simulink model "lab4"  (R2018a)
settings: Solver=FixedStepDiscrete  StartTime=0  StopTime=0.2  RelTol=1e-3
libraries: powerlib x12, electricdrivelib x1
settings Model: Creator=Ali  LastModifiedBy=Ali

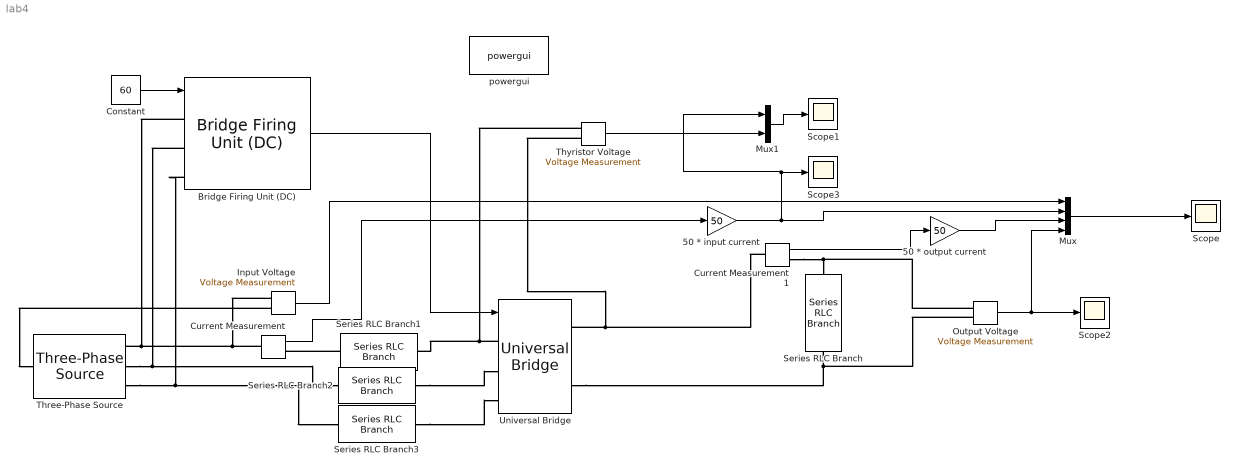
== system lab4 ==
  "50 * input current " : Gain  Gain=50
  50 * output current : Gain  Gain=50
  Bridge Firing Unit (DC) : electricdrivelib/Fundamental Drive Blocks/Bridge Firing Unit (DC)  OverrideUsingVariant=AC_Detailed_two quadrant  detailLevel=Detailed  nbPhases=3  numQuad=2  x4=50  x9=10  Ts=2e-6
      settings: SourceProductName=Simscape Power Systems  SourceProductBaseCode=PS
  Constant : Constant  Value=60
  Current Measurement : powerlib/Measurements/Current Measurement  PhasorSimulation=off  OutputType=Complex  PSBequivalent=0
  Current Measurement1 : powerlib/Measurements/Current Measurement  PhasorSimulation=off  OutputType=Complex  PSBequivalent=0
  Input Voltage : powerlib/Measurements/Voltage Measurement  PhasorSimulation=off  OutputType=Complex  PSBequivalent=0
  Mux : Mux
  Mux1 : Mux  Inputs=2
  Output Voltage : powerlib/Measurements/Voltage Measurement  PhasorSimulation=off  OutputType=Complex  PSBequivalent=0
  Scope{,1..3} (4 alike) : Scope
  Series RLC Branch : powerlib/Elements/Series RLC Branch  LConnTagsString=__new0  RConnTagsString=__new0  BranchType=RL  Resistance=72  Inductance=0.4575  SetiL0=off  InitialCurrent=0  Capacitance=1e-6  Setx0=off  InitialVoltage=0  Measurements=None
  Series RLC Branch1 : powerlib/Elements/Series RLC Branch  LConnTagsString=__new0  RConnTagsString=__new0  BranchType=L  Resistance=72  Inductance=5e-3  SetiL0=off  InitialCurrent=0  Capacitance=1e-6  Setx0=off  InitialVoltage=0  Measurements=None
  Series RLC Branch2 : powerlib/Elements/Series RLC Branch  LConnTagsString=__new0  RConnTagsString=__new0  BranchType=L  Resistance=72  Inductance=5e-3  SetiL0=off  InitialCurrent=0  Capacitance=1e-6  Setx0=off  InitialVoltage=0  Measurements=None
  Series RLC Branch3 : powerlib/Elements/Series RLC Branch  LConnTagsString=__new0  RConnTagsString=__new0  BranchType=L  Resistance=72  Inductance=5e-3  SetiL0=off  InitialCurrent=0  Capacitance=1e-6  Setx0=off  InitialVoltage=0  Measurements=None
  Three-Phase Source : powerlib/Electrical Sources/Three-Phase Source  InternalConnection=Yn  VoltagePhases=off  Voltage=347  PhaseAngle=0  Voltage_phases=[25e3 25e3 25e3]/sqrt(3)  PhaseAngles_phases=[0 -120 +120]  Frequency=50  NonIdealSource=on  SpecifyImpedance=off  Resistance=0  Inductance=0  ShortCircuitLevel=100e6  BaseVoltage=0  XRratio=7  BusType=swing  Pref=10e3  Qref=0  Prefabc=[10e3, 10e3, 10e3]  Qrefabc=[0, 0, 0]  Qmin=-inf  Qmax=inf
  Thyristor Voltage : powerlib/Measurements/Voltage Measurement  PhasorSimulation=off  OutputType=Complex  PSBequivalent=0
  Universal Bridge : powerlib/Power Electronics/Universal Bridge  Arms=3  SnubberResistance=1e5  SnubberCapacitance=inf  Device=Thyristors  Ron=1e-3  Lon=0  ForwardVoltages="[  0  0  ]"  ForwardVoltage=0  GTOparameters=[ 10e-6 , 20e-6 ]  IGBTparameters=[ 1e-6 , 2e-6 ]  Measurements=None  Measurements_2=None  converterType=Rectifier
  powergui : powerlib/powergui  Priority=1  SimulationMode=Discrete  SampleTime=50e-6  frequency=60  Iterations=50  frequencyindice=50  Pbase=100e6  ErrMax=1e-4  UnitsV=kV  UnitsW=MW  buscounter=0  FunctionMessages=off  echomessages=off  EnableUseOfTLC=off  CurrentSourceSwitches=off  DisableSnubberDevices=off  DisableRonSwitches=off  DisableVfSwitches=off  DisplayEquations=off  SolverType=Tustin/Backward Euler (TBE)  Interpol=off  ExternalGateDelay=off  methode=off  Ts=100  x0status=blocks  SPID=on  SwTol=0  HookPort=off  RestoreLinks=warning  ResistiveCurrentMeasurement=off  Frange=[0:2:500]  Ylog=off  Xlog=on  ShowGrid=off  save=off  variable=ZData  structure=0  ZoomFFT=off  StartTime=0.0  cycles=1  DisplayStyle=1  fundamental=60  FreqAxis=off  MaxFrequency=1000  frequencyindicesteady=1  RmsSteady=1  display=off
  wires:
  Mux/1 -> Scope/1
  Output Voltage/1 -> Scope2/1, Mux/4
  Current Measurement1/1 -> 50 * output current/1
  Current Measurement/1 -> "50 * input current "/1
  Input Voltage/1 -> Mux/1
  "50 * input current "/1 -> Mux1/1, Scope3/1, Mux/2
  50 * output current/1 -> Mux/3
  Constant/1 -> Bridge Firing Unit (DC)/1
  Bridge Firing Unit (DC)/1 -> Universal Bridge/1
  Mux1/1 -> Scope1/1
  Thyristor Voltage/1 -> Mux1/2
  connections:
  Current Measurement/LConn1 -- Input Voltage/LConn1 -- Bridge Firing Unit (DC)/LConn1 -- Three-Phase Source/RConn1
  Output Voltage/LConn2 -- Universal Bridge/RConn2 -- Series RLC Branch/RConn1
  Output Voltage/LConn1 -- Current Measurement1/RConn1 -- Series RLC Branch/LConn1
  Input Voltage/LConn2 -- Three-Phase Source/LConn1
  Universal Bridge/LConn1 -- Series RLC Branch1/LConn1 -- Thyristor Voltage/LConn1
  Three-Phase Source/RConn2 -- Series RLC Branch2/RConn1 -- Bridge Firing Unit (DC)/LConn2
  Three-Phase Source/RConn3 -- Series RLC Branch3/RConn1 -- Bridge Firing Unit (DC)/LConn3
  Current Measurement1/LConn1 -- Thyristor Voltage/LConn2 -- Universal Bridge/RConn1
  Series RLC Branch1/RConn1 -- Current Measurement/RConn1
  Series RLC Branch2/LConn1 -- Universal Bridge/LConn2
  Series RLC Branch3/LConn1 -- Universal Bridge/LConn3
